simulink model "FaultModel"  (R2020b)
settings: Solver=ode4  StartTime=0.0  StopTime=inf  FixedStep=0.001  RelTol=1e-3
PreLoadFcn:
  | filepath  = fileparts(get_param(bdroot, 'FileName'));
  | cd(filepath);
InitFcn:
  | Init
undefined symbols (not defined in the file): d_i, Earth, F, h_i, Light, MIL, ModelFailEnable, ModelInit_RPM, ModelParam_BattHoverMinutes, ModelParam_BattHoverThr, ModelParam_envAltitude, ModelParam_GPSEphFinal, ModelParam_GPSEpvFinal, ModelParam_GPSEpvInitial, ModelParam_GPSEpvTimeConstant, ModelParam_GPSFix3DFix, ModelParam_GPSSatsVisible, ModelParam_motorCr, ModelParam_motorJm, ModelParam_motorMinThr, ModelParam_motorT, ModelParam_motorWb, ModelParam_noiseGPSSampTime, ModelParam_noiseLowPassFilterCoeAccel, ModelParam_noiseLowPassFilterCoeGyro, ModelParam_noisePowerIMU, ModelParam_noisePowerOffGainAccel, ModelParam_noisePowerOffGainAccelZ, ModelParam_noisePowerOffGainGyro, ModelParam_noisePowerOffGainGyroZ, ModelParam_noisePowerOffGainMag, ModelParam_noisePowerOffGainMagZ, ModelParam_noisePowerOnGainAccel, ModelParam_noisePowerOnGainAccelZ, ModelParam_noisePowerOnGainGyro, ModelParam_noisePowerOnGainGyroZ, ModelParam_noisePowerOnGainMag, ModelParam_noisePowerOnGainMagZ, ModelParam_noiseSampleTimeAccel, ModelParam_noiseSampleTimeGyro, ModelParam_noiseSampleTimeMag, ModelParam_rotorCm, ModelParam_rotorCt, ModelParam_timeSampBaro, ModelParam_uavCCm, ModelParam_uavCd, ModelParam_uavDearo, ModelParam_uavJ, ModelParam_uavMass, ModelParam_uavMotNumbs, ModelParam_uavR, ModelParam_uavType, Moderate, Newton, Raphson, WGS84
libraries: simulink x12, aerolibwind2 x3, aerolibtransform2 x3, sharedtransform x3, aerolibasang x3, aerolibatmos2 x2, aerolibutil x2, shared6dof x1, aerolibconvert2 x1, aerolibobsolete x1, aerolibnav x1, aerolibgravity2 x1
(part 1 of 4)
settings Model: Creator=Jinrui  LastModifiedBy=DELL
settings DataIOCC: ReturnWorkspaceOutputs=off
settings OptimizationCC: ZeroExternalMemoryAtStartup=off  ZeroInternalMemoryAtStartup=off  EfficientTunableParamExpr=on
settings DebuggingCC: ParameterTunabilityLossMsg=error  ArithmeticOperatorsInVariantConditions=warning
settings SFSimCC: SimUseLocalCustomCode=off  MATLABDynamicMemAlloc=off  CustomCodeUndefinedFunction=UseInterfaceOnly  SimTargetLang=C++
settings RTWCC: Description=Embedded Coder  SystemTargetFile=ert.tlc  GenerateMakefile=off  PackageGeneratedCodeAndArtifacts=on  PackageName=MulticopterModel  TemplateMakefile=ert_default_tmf  RTWUseLocalCustomCode=off  TargetLang=C++  RTWCompilerOptimization=on
settings CodeAppCC: ForceParamTrailComments=on  OperatorAnnotations=on  SimulinkDataObjDesc=on  SFDataObjDesc=on  MATLABFcnDesc=on  InsertBlockDesc=on  StateflowObjectComments=on  MATLABSourceComments=on
settings ERTTargetCC: TargetLangStandard=C++03 (ISO)  MultiwordLength=2048  GenerateSampleERTMain=on  CodeInterfacePackaging=C++ class  SupportContinuousTime=on  MultiInstanceErrorCode=None  RootIOFormat=Structure reference  ERTCustomFileTemplate=example_file_process.tlc  ERTFilePackagingFormat=Compact
settings SimscapeCC: SimscapeNormalizeSystem=off

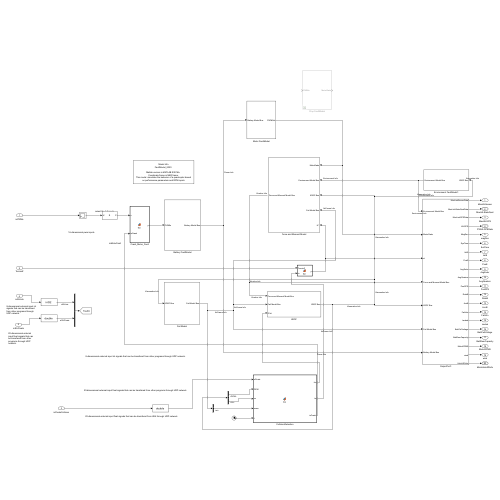
[thumbnail: Simulink's stored preview of the top-level diagram]
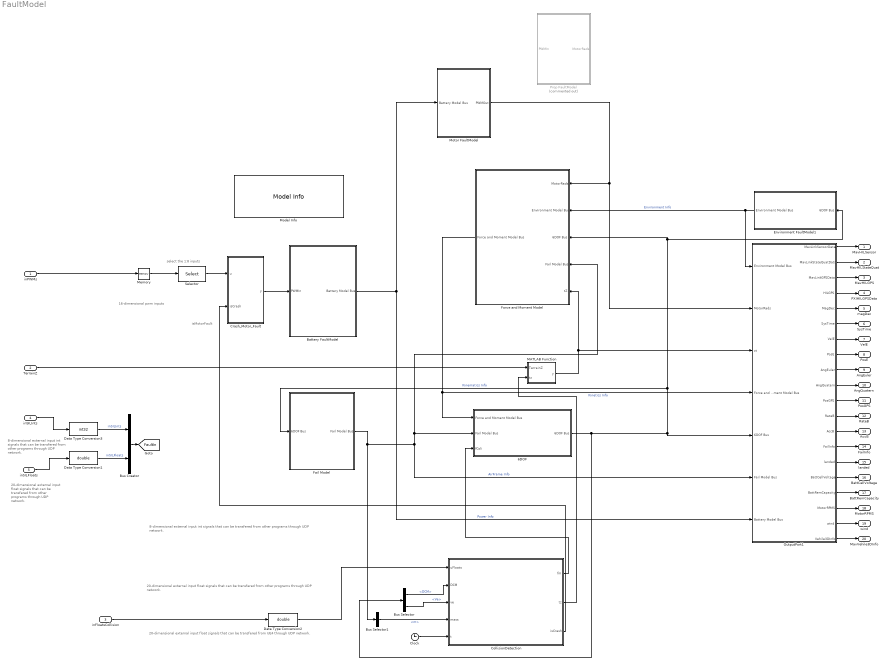
== system FaultModel ==
  note: 16-dimensional pwm inputs
  note: 20-dimensional external input float signals that can be transfered from UE4 through UDP network.
  note: select the 1:8 inputs
  note: 8-dimensional external input int signals that can be transfered from other programs through UDP network.
  note: 20-dimensional external input float signals that can be transfered from other programs through UDP network.
  note: isMotorFault
  note: 20-dimensional external input float signals that can be transfered from other programs through UDP network.
  note: 8-dimensional external input int signals that can be transfered from other programs through UDP network.
  inPWMs : Inport  PortDimensions=8
  TerrainZ : Inport  Port=2  PortDimensions=1
  inFloatsCollision : Inport  Port=3  OutDataTypeStr=single  PortDimensions=20
  inSILInts : Inport  Port=4  OutDataTypeStr=int32  PortDimensions=8
  inSILFloats : Inport  Port=5  OutDataTypeStr=single  PortDimensions=20
  6DOF : Subsystem
  Battery FaultModel : Subsystem
  Bus Creator : BusCreator  Inputs=2
  Bus Selector : BusSelector  OutputSignals=DCM,Ve
  Bus Selector1 : BusSelector  OutputSignals=m
  Clock : Clock
  CollisionDetection : MATLAB Function  TreatAsAtomicUnit=on
  Crash_Motor_Fault : MATLAB Function  TreatAsAtomicUnit=on
  Data Type Conversion1 : DataTypeConversion  OutDataTypeStr=double
  Data Type Conversion2 : DataTypeConversion  OutDataTypeStr=double
  Data Type Conversion3 : DataTypeConversion  OutDataTypeStr=int32
  Environment FaultModel1 : Subsystem
  Fail Model : Subsystem
  Force and Moment Model : Subsystem
  MATLAB Function : MATLAB Function  TreatAsAtomicUnit=on
  Memory : Memory
  Model Info : simulink/Model-Wide Utilities/Model Info  Frame=on  DisplayStringWithTags=|  HorizontalTextAlignment=Center  LeftAlignmentValue=0.5
      | Model Info
      | %<ModelName> 
      | %<Description>   
      | Matlab version is MATLAB R2016b. 
      | Coordinate frame is NED frame.
      |  This model  simulates the behavior of a quadcopter based 
      | on performance parameters and RPM inputs
  Motor FaultModel : Subsystem
  OutputPort1 : Subsystem
  Prop FaultModel : Subsystem  Commented=on
  Selector : Selector  InputPortWidth=8  IndexOptions=Index vector (dialog)  Indices=[1:8]  OutputSizes=1
  MavHILSensor : Outport
  MavHILStateQuat : Outport  Port=2  OutDataTypeStr=Bus: MavLinkStateQuat  VectorParamsAs1DForOutWhenUnconnected=off
  MavHILGPS : Outport  Port=3
  PXIHILGPSData : Outport  Port=4  OutDataTypeStr=Bus: HILGPS  VectorParamsAs1DForOutWhenUnconnected=off
  magDec : Outport  Port=5  VectorParamsAs1DForOutWhenUnconnected=off
  SysTime : Outport  Port=6  VectorParamsAs1DForOutWhenUnconnected=off
  VelE : Outport  Port=7  VectorParamsAs1DForOutWhenUnconnected=off
  PosE : Outport  Port=8  VectorParamsAs1DForOutWhenUnconnected=off
  AngEuler : Outport  Port=9  VectorParamsAs1DForOutWhenUnconnected=off
  AngQuatern : Outport  Port=10  VectorParamsAs1DForOutWhenUnconnected=off
  PosGPS : Outport  Port=11  VectorParamsAs1DForOutWhenUnconnected=off
  RateB : Outport  Port=12  VectorParamsAs1DForOutWhenUnconnected=off
  AccB : Outport  Port=13  VectorParamsAs1DForOutWhenUnconnected=off
  FailInfo : Outport  Port=14  VectorParamsAs1DForOutWhenUnconnected=off
  landed : Outport  Port=15  VectorParamsAs1DForOutWhenUnconnected=off
  BattCellVoltage : Outport  Port=16  VectorParamsAs1DForOutWhenUnconnected=off
  BattRemCapacity : Outport  Port=17  VectorParamsAs1DForOutWhenUnconnected=off
  MotorRPMS : Outport  Port=18  VectorParamsAs1DForOutWhenUnconnected=off
  wind : Outport  Port=19  VectorParamsAs1DForOutWhenUnconnected=off
  MavVehile3DInfo : Outport  Port=20  OutDataTypeStr=Bus: MavVehileInfo  VectorParamsAs1DForOutWhenUnconnected=off
  tag scope: FaultIn=global
  wires:
  OutputPort1/14(FailInfo) -> FailInfo/1
  OutputPort1/9(AngEuler) -> AngEuler/1
  OutputPort1/17(BattRemCapacity) -> BattRemCapacity/1
  Memory/1 -> Selector/1
  OutputPort1/1(MavLinkSensorData) -> MavHILSensor/1
  Force and Moment Model/1(Force and Moment Model Bus) -> 6DOF/1(Force and Moment Model Bus), OutputPort1/4(Force and Moment Model Bus)  "Kinetics Info"
  Battery FaultModel/1(Battery Model Bus) -> Motor FaultModel/1(Battery Model Bus), OutputPort1/7(Battery Model Bus)  "Power Info"
  Fail Model/1(Fail Model Bus) -> Bus Selector1/1, Force and Moment Model/4(Fail Model Bus), 6DOF/2(Fail Model Bus), OutputPort1/6(Fail Model Bus)  "AirFrame Info"
  Bus Selector1/1 -> CollisionDetection/4(mass)  "<m>"
  OutputPort1/15(landed) -> landed/1
  TerrainZ/1 -> MATLAB Function/1(TerrainZ)
  OutputPort1/8(PosE) -> PosE/1
  OutputPort1/19(wind) -> wind/1
  Environment FaultModel1/1(Environment Model Bus) -> OutputPort1/1(Environment Model Bus), Force and Moment Model/2(Environment Model Bus)  "Environment Info"
  inFloatsCollision/1 -> Data Type Conversion2/1
  Bus Selector/1 -> CollisionDetection/2(DCM)  "<DCM>"
  inPWMs/1 -> Memory/1
  MATLAB Function/1(y) -> Force and Moment Model/5("tZ "), OutputPort1/3(zt)
  CollisionDetection/2(tz) -> MATLAB Function/2(tz)
  OutputPort1/10(AngQuatern) -> AngQuatern/1
  OutputPort1/7(VelE) -> VelE/1
  OutputPort1/13(AccB) -> AccB/1
  6DOF/1(6DOF Bus) -> Bus Selector/1, Force and Moment Model/3(6DOF Bus), Environment FaultModel1/1(6DOF Bus), Fail Model/1(6DOF Bus), OutputPort1/5(6DOF Bus)  "Kinematics Info"
  OutputPort1/12(RateB) -> RateB/1
  OutputPort1/5(MagDec) -> magDec/1
  CollisionDetection/1(fm) -> 6DOF/3(fColi)
  OutputPort1/18(MotorRPMS) -> MotorRPMS/1
  OutputPort1/16(BattCellVoltage) -> BattCellVoltage/1
  OutputPort1/20(Vehile3DInfo) -> MavVehile3DInfo/1
  CollisionDetection/3(isCrash) -> Crash_Motor_Fault/2(isCrash)
  Bus Selector/2 -> CollisionDetection/3(ve)  "<Ve>"
  OutputPort1/2(MavLinkStateQuatData) -> MavHILStateQuat/1
  OutputPort1/3(MavLinkGPSData) -> MavHILGPS/1
  Data Type Conversion2/1 -> CollisionDetection/1(uFloats)
  OutputPort1/6(SysTime) -> SysTime/1
  OutputPort1/4(HILGPS) -> PXIHILGPSData/1
  OutputPort1/11(PosGPS) -> PosGPS/1
  Clock/1 -> CollisionDetection/5(t)
  Selector/1 -> Crash_Motor_Fault/1(u)
  Data Type Conversion3/1 -> Bus Creator/1  "inSILInts"
  inSILFloats/1 -> Data Type Conversion1/1
  inSILInts/1 -> Data Type Conversion3/1
  Data Type Conversion1/1 -> Bus Creator/2  "inSILFloats"
  Bus Creator/1 -> [FaultIn]
  Crash_Motor_Fault/1(y) -> Battery FaultModel/1(PWMIn)
  Motor FaultModel/1(PWMOut) -> OutputPort1/2(MotorRads), Force and Moment Model/1(MotorRads)

== system FaultModel/6DOF ==
  Force and Moment Model Bus : Inport
  Fail Model Bus : Inport  Port=2
  fColi : Inport  Port=3
  Bus Creator : BusCreator  Inputs=8
  Bus Selector : BusSelector  OutputSignals=dM,m,J
  Bus Selector1 : BusSelector  OutputSignals=Fb,Mb
  Constant_dI/dt : Constant  Value=zeros(3,3)
  Custom Variable Mass 6DOF (Quaternion) : shared6dof/6DOF (Euler Angles)  units=Metric (MKS)  mtype=Custom Variable  rep=Quaternion  xme_0=ModelInit_PosE  Vm_0=ModelInit_VelB  eul_0=ModelInit_AngEuler  pm_0=ModelInit_RateB  mass_0=1.0  mass_e=0.5  mass_f=2.0  inertia=eye(3)  inertia_e=eye(3)  inertia_f=2*eye(3)  k_quat=1.0  vre_flag=off  abi_flag=off  aMode=aMode  xme_statename=''  Vm_statename=''  eul_statename=''  quat_statename=''  pm_statename=''  mass_statename=''
      settings: SourceProductBaseCode=AE,PW,MT,UV,VE,VP
  Demux : Demux  Outputs=2
  Sum : Sum  Inputs=+++
  Sum1 : Sum  Inputs=++|
  6DOF Bus : Outport  VectorParamsAs1DForOutWhenUnconnected=off
  wires:
  Bus Selector1/1 -> Sum1/2  "<Fb>"
  Bus Selector/2 -> Custom Variable Mass 6DOF (Quaternion)/3  "<m>"
  Custom Variable Mass 6DOF (Quaternion)/8 -> Bus Creator/8  "AccB"
  Sum/1 -> Custom Variable Mass 6DOF (Quaternion)/2
  Constant_dI/dt/1 -> Custom Variable Mass 6DOF (Quaternion)/4
  Custom Variable Mass 6DOF (Quaternion)/5 -> Bus Creator/5  "Vb"
  Custom Variable Mass 6DOF (Quaternion)/6 -> Bus Creator/6  "wb"
  Custom Variable Mass 6DOF (Quaternion)/1 -> Bus Creator/1  "Ve"
  Custom Variable Mass 6DOF (Quaternion)/4 -> Bus Creator/4  "DCM"
  Custom Variable Mass 6DOF (Quaternion)/2 -> Bus Creator/2  "Xe"
  Custom Variable Mass 6DOF (Quaternion)/3 -> Bus Creator/3  "Eular(rad)"
  Custom Variable Mass 6DOF (Quaternion)/7 -> Bus Creator/7  "dwb/dt"
  Bus Selector/3 -> Custom Variable Mass 6DOF (Quaternion)/5  "<J>"
  Bus Selector/1 -> Sum/2  "<dM>"
  Bus Selector1/2 -> Sum/1  "<Mb>"
  Fail Model Bus/1 -> Bus Selector/1
  Force and Moment Model Bus/1 -> Bus Selector1/1
  Bus Creator/1 -> 6DOF Bus/1
  Sum1/1 -> Custom Variable Mass 6DOF (Quaternion)/1
  Demux/1 -> Sum1/1
  fColi/1 -> Demux/1
  Demux/2 -> Sum/3

== system FaultModel/Battery FaultModel ==
  PWMIn : Inport
  FaultModelTmp : Subsystem
  Battery Model Bus : Outport  VectorParamsAs1DForOutWhenUnconnected=off
  wires:
  [FaultIn] -> FaultModelTmp/1(FaultIn)
  PWMIn/1 -> FaultModelTmp/2(PWMIn)
  FaultModelTmp/1(Battery Model Bus) -> Battery Model Bus/1

== system FaultModel/Environment FaultModel1 ==
  6DOF Bus : Inport
  Env FaultWindModel : Subsystem
  Environment Model Bus : Outport  VectorParamsAs1DForOutWhenUnconnected=off
  wires:
  6DOF Bus/1 -> Env FaultWindModel/1(6DOF Bus)
  [FaultIn] -> Env FaultWindModel/2(FaultIn)
  Env FaultWindModel/1(Environment Model Bus) -> Environment Model Bus/1

== system FaultModel/Fail Model ==
  6DOF Bus : Inport
  Prop FaultModel : Subsystem
  Fail Model Bus : Outport  VectorParamsAs1DForOutWhenUnconnected=off
  wires:
  [FaultIn] -> Prop FaultModel/1(FaultIn)
  Prop FaultModel/1(Fail Model Bus) -> Fail Model Bus/1
  6DOF Bus/1 -> Prop FaultModel/2(6DOF Bus)

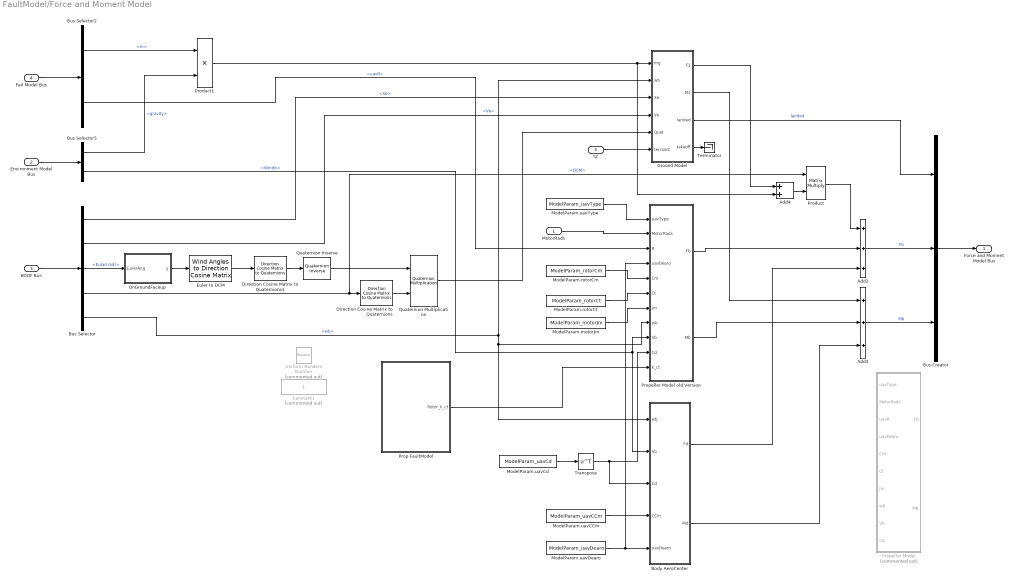
== system FaultModel/Force and Moment Model ==
  MotorRads : Inport
  Environment Model Bus : Inport  Port=2
  6DOF Bus : Inport  Port=3
  Fail Model Bus : Inport  Port=4
  "tZ " : Inport  Port=5
  Add2 : Sum  Inputs=+++
  Add3 : Sum  Inputs=+++
  Add4 : Sum
  Body AeroCenter : MATLAB Function  TreatAsAtomicUnit=on
  Bus Creator : BusCreator  Inputs=3
  Bus Selector : BusSelector  OutputSignals=Xe,Ve,Eular(rad),DCM,wb
  Bus Selector2 : BusSelector  OutputSignals=m,uavR
  Bus Selector5 : BusSelector  OutputSignals=gravity,Windb
  Constant1 : Constant  Commented=on
  Direction Cosine Matrix to Quaternions : sharedtransform/Direction Cosine Matrix  to Quaternions  aMode=aMode  action=None  tolerance=eps(2)
      settings: SourceProductBaseCode=AE,PW,MT,UV,VE,VP
  Direction Cosine Matrix to Quaternions1 : sharedtransform/Direction Cosine Matrix  to Quaternions  aMode=aMode  action=None  tolerance=eps(2)
      settings: SourceProductBaseCode=AE,PW,MT,UV,VE,VP
  Euler to DCM : aerolibtransform2/Wind Angles to  Direction Cosine Matrix
      settings: SourceProductBaseCode=AE
  Ground Model : MATLAB Function  TreatAsAtomicUnit=on
  ModelParam.motorJm : Constant  Value=ModelParam_motorJm
  ModelParam.rotorCm : Constant  Value=ModelParam_rotorCm
  ModelParam.rotorCt : Constant  Value=ModelParam_rotorCt
  ModelParam.uavCCm : Constant  Value=ModelParam_uavCCm
  ModelParam.uavCd : Constant  Value=ModelParam_uavCd
  ModelParam.uavDearo : Constant  Value=ModelParam_uavDearo
  ModelParam.uavType : Constant  Value=ModelParam_uavType
  OnGroundFaceup : MATLAB Function  TreatAsAtomicUnit=on
  Product : Product  Multiplication=Matrix(*)
  Product1 : Product
  Prop FaultModel : Subsystem
  Propeller Model : Subsystem  Commented=on  TreatAsAtomicUnit=on
  Propeller Model old Version : MATLAB Function  TreatAsAtomicUnit=on
  Quaternion Inverse : aerolibutil/Quaternion Inverse
  Quaternion Multiplication : aerolibutil/Quaternion Multiplication
  Terminator : Terminator
  Transpose : Math  Operator=transpose  SignedPower=on  SaturateOnIntegerOverflow=on
  Uniform Random Number : UniformRandomNumber  Commented=on  Minimum=[-1,-1,-1]  Maximum=[1,1,1]  Seed=[145787,351545,2864]  SampleTime=0.05
  Force and Moment Model Bus : Outport  VectorParamsAs1DForOutWhenUnconnected=off
  wires:
  Body AeroCenter/2(Md) -> Add3/3
  Body AeroCenter/1(Fd) -> Add2/3
  Propeller Model old Version/2(Mb) -> Add3/2
  Propeller Model old Version/1(Fb) -> Add2/2
  Ground Model/4(takeoff) -> Terminator/1
  Ground Model/3(landed) -> Bus Creator/1  "landed"
  "tZ "/1 -> Ground Model/6(terrainZ)
  Add3/1 -> Bus Creator/3  "Mb"
  Add2/1 -> Bus Creator/2  "Fb"
  ModelParam.uavType/1 -> Propeller Model old Version/1(uavType)
  Quaternion Multiplication/1 -> Ground Model/5(Quet)
  Quaternion Inverse/1 -> Quaternion Multiplication/1
  Direction Cosine Matrix to Quaternions1/1 -> Quaternion Inverse/1
  Euler to DCM/1 -> Direction Cosine Matrix to Quaternions1/1
  OnGroundFaceup/1(y) -> Euler to DCM/1
  Direction Cosine Matrix to Quaternions/1 -> Quaternion Multiplication/2
  ModelParam.rotorCt/1 -> Propeller Model old Version/6(Ct)
  Product/1 -> Add2/1
  Ground Model/1(F1) -> Add4/1
  Add4/1 -> Product/2
  Product1/1 -> Ground Model/1(mg), Add4/2
  Ground Model/2(M1) -> Add3/1
  Bus Selector/4 -> Direction Cosine Matrix to Quaternions/1, Product/1  "<DCM>"
  ModelParam.motorJm/1 -> Propeller Model old Version/7(Jm)
  ModelParam.rotorCm/1 -> Propeller Model old Version/5(Cm)
  MotorRads/1 -> Propeller Model old Version/2(MotorRads)
  Bus Selector/5 -> Propeller Model old Version/8(wb), Body AeroCenter/1(wb), Ground Model/2(wb)  "<wb>"
  ModelParam.uavCCm/1 -> Body AeroCenter/4(CCm)
  Bus Creator/1 -> Force and Moment Model Bus/1
  6DOF Bus/1 -> Bus Selector/1
  Bus Selector/2 -> Ground Model/4(Ve)  "<Ve>"
  Bus Selector/1 -> Ground Model/3(Xe)  "<Xe>"
  Bus Selector/3 -> OnGroundFaceup/1(EulerAng)  "<Eular(rad)>"
  Bus Selector2/1 -> Product1/1  "<m>"
  Bus Selector5/1 -> Product1/2  "<gravity>"
  Fail Model Bus/1 -> Bus Selector2/1
  Environment Model Bus/1 -> Bus Selector5/1
  Bus Selector2/2 -> Propeller Model old Version/3(R)  "<uavR>"
  Bus Selector5/2 -> Body AeroCenter/2(Vb), Propeller Model old Version/9(Vb)  "<Windb>"
  ModelParam.uavDearo/1 -> Propeller Model old Version/4(uavDearo), Body AeroCenter/5(uavDearo)
  ModelParam.uavCd/1 -> Transpose/1
  Transpose/1 -> Body AeroCenter/3(Cd), Propeller Model old Version/10(Cd)
  Prop FaultModel/1(Rotor_k_ct) -> Propeller Model old Version/11(k_ct)

== system FaultModel/Motor FaultModel ==
  Battery Model Bus : Inport
  Bus Selector : BusSelector  OutputSignals=PWMOut
  FaultModelTmp : Subsystem
  PWMOut : Outport
  wires:
  Battery Model Bus/1 -> Bus Selector/1
  [FaultIn] -> FaultModelTmp/1(FaultIn)
  FaultModelTmp/1(PWMOut) -> PWMOut/1
  Bus Selector/1 -> FaultModelTmp/2(PWMIn)  "<PWMOut>"

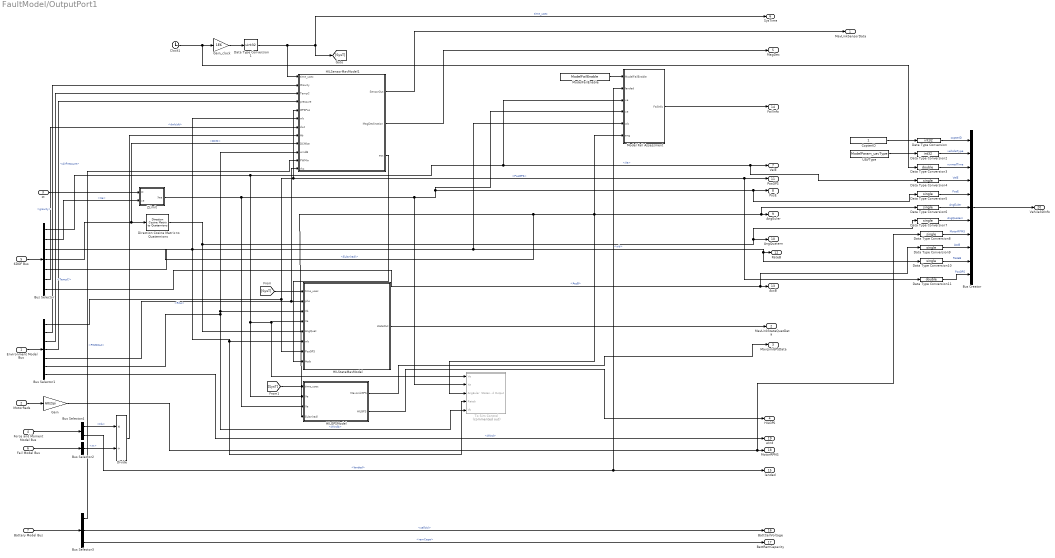
== system FaultModel/OutputPort1 ==
  Environment Model Bus : Inport
  MotorRads : Inport  Port=2
  zt : Inport  Port=3
  Force and Moment Model Bus : Inport  Port=4
  6DOF Bus : Inport  Port=5
  Fail Model Bus : Inport  Port=6
  Battery Model Bus : Inport  Port=7
  Bus Creator : BusCreator  Inputs=11  OutDataTypeStr=Bus: MavVehileInfo
  Bus Selector : BusSelector  OutputSignals=Ve,Xe,Eular(rad),DCM,wb,dwb/dt,AccB
  Bus Selector1 : BusSelector  OutputSignals=PosGPS,gravity,TempC,AirPressure,Rho,Windb,Wind
  Bus Selector2 : BusSelector  OutputSignals=m
  Bus Selector3 : BusSelector  OutputSignals=PWMOut,cellVol,remCapa
  Bus Selector4 : BusSelector  OutputSignals=Fb,landed
  Clock1 : Clock
  CopterID : Constant
  Data Type Conversion : DataTypeConversion  OutDataTypeStr=int32
  Data Type Conversion1 : DataTypeConversion  OutDataTypeStr=uint32
  Data Type Conversion{4..10} (7 alike) : DataTypeConversion  OutDataTypeStr=single
  Data Type Conversion11 : DataTypeConversion  OutDataTypeStr=double
  Data Type Conversion2 : DataTypeConversion  OutDataTypeStr=int32
  Data Type Conversion3 : DataTypeConversion  OutDataTypeStr=double
  Direction Cosine Matrix to Quaternions : sharedtransform/Direction Cosine Matrix  to Quaternions  aMode=aMode  action=None  tolerance=eps(2)
      settings: SourceProductBaseCode=AE,PW,MT,UV,VE,VP
  Divide : Product  Inputs=*/
  Gain : Gain  Gain=60/2/pi
  Gain_clock : Gain  Gain=1E6
  HILGPSModel : Subsystem
  HILSensorMavModel1 : Subsystem
  HILStateMavModel : Subsystem
  Model Fail Assessment : MATLAB Function  TreatAsAtomicUnit=on
  ModelFailEnable : Constant  Value=ModelFailEnable
  To Sim Control : Subsystem  Commented=on
  UAVType : Constant  Value=ModelParam_uavType
  ZLimit : MATLAB Function  TreatAsAtomicUnit=on
  MavLinkSensorData : Outport  VectorParamsAs1DForOutWhenUnconnected=off
  MavLinkStateQuatData : Outport  Port=2  VectorParamsAs1DForOutWhenUnconnected=off
  MavLinkGPSData : Outport  Port=3  VectorParamsAs1DForOutWhenUnconnected=off
  HILGPS : Outport  Port=4  VectorParamsAs1DForOutWhenUnconnected=off
  MagDec : Outport  Port=5  VectorParamsAs1DForOutWhenUnconnected=off
  SysTime : Outport  Port=6  VectorParamsAs1DForOutWhenUnconnected=off
  VelE : Outport  Port=7  VectorParamsAs1DForOutWhenUnconnected=off
  PosE : Outport  Port=8  VectorParamsAs1DForOutWhenUnconnected=off
  AngEuler : Outport  Port=9  VectorParamsAs1DForOutWhenUnconnected=off
  AngQuatern : Outport  Port=10  VectorParamsAs1DForOutWhenUnconnected=off
  PosGPS : Outport  Port=11  VectorParamsAs1DForOutWhenUnconnected=off
  RateB : Outport  Port=12  VectorParamsAs1DForOutWhenUnconnected=off
  AccB : Outport  Port=13  VectorParamsAs1DForOutWhenUnconnected=off
  FailInfo : Outport  Port=14  VectorParamsAs1DForOutWhenUnconnected=off
  landed : Outport  Port=15  VectorParamsAs1DForOutWhenUnconnected=off
  BattCellVoltage : Outport  Port=16  VectorParamsAs1DForOutWhenUnconnected=off
  BattRemCapacity : Outport  Port=17  VectorParamsAs1DForOutWhenUnconnected=off
  MotorRPMS : Outport  Port=18  VectorParamsAs1DForOutWhenUnconnected=off
  wind : Outport  Port=19  VectorParamsAs1DForOutWhenUnconnected=off
  Vehile3DInfo : Outport  Port=20  VectorParamsAs1DForOutWhenUnconnected=off
  wires:
  [SysT] -> HILGPSModel/1(time_usec)
  [SysT] -> HILStateMavModel/1(time_usec)
  Bus Selector/5 -> HILSensorMavModel1/6(wb), Data Type Conversion10/1, RateB/1, Model Fail Assessment/5(wb), To Sim Control/4(Rateb), HILStateMavModel/6(wb)  "<wb>"
  Bus Selector/4 -> HILSensorMavModel1/9(DCMbe), Direction Cosine Matrix to Quaternions/1  "<DCM>"
  Bus Selector/1 -> HILGPSModel/2(Ve), To Sim Control/1(Ve), HILStateMavModel/4(Ve), Model Fail Assessment/3(ve), Data Type Conversion4/1, VelE/1  "<Ve>"
  Bus Selector/6 -> HILSensorMavModel1/7(dwt)  "<dwb/dt>"
  Bus Selector/3 -> Data Type Conversion6/1, AngEuler/1, Model Fail Assessment/6(ang), To Sim Control/3(AngEuler), HILGPSModel/4(Eular(rad))  "<Eular(rad)>"
  Clock1/1 -> Data Type Conversion3/1, Gain_clock/1
  Data Type Conversion1/1 -> HILSensorMavModel1/1(time_usec), SysTime/1, [SysT]  "time_usec"
  Gain_clock/1 -> Data Type Conversion1/1
  6DOF Bus/1 -> Bus Selector/1
  zt/1 -> ZLimit/1(zt)
  Bus Selector/2 -> ZLimit/2(xe)  "<Xe>"
  Environment Model Bus/1 -> Bus Selector1/1
  Bus Selector1/1 -> HILStateMavModel/7(PosGPS), HILSensorMavModel1/5(GPSPos), Data Type Conversion11/1, PosGPS/1  "<PosGPS>"
  Bus Selector1/2 -> HILSensorMavModel1/2(Gravity)  "<gravity>"
  Bus Selector1/3 -> HILSensorMavModel1/3(TempC)  "<TempC>"
  Bus Selector1/4 -> HILSensorMavModel1/4(pressure)  "<AirPressure>"
  Bus Selector1/5 -> HILSensorMavModel1/12(rho), HILStateMavModel/2(pho)  "<Rho>"
  Bus Selector1/6 -> HILSensorMavModel1/10(windB), HILStateMavModel/3(Vb), To Sim Control/5(Vb)  "<Windb>"
  Bus Selector2/1 -> Divide/2  "<m>"
  Bus Selector4/1 -> Divide/1  "<Fb>"
  Force and Moment Model Bus/1 -> Bus Selector4/1
  Fail Model Bus/1 -> Bus Selector2/1
  Bus Selector4/2 -> landed/1, Model Fail Assessment/2(landed)  "<landed>"
  Battery Model Bus/1 -> Bus Selector3/1
  Bus Selector3/2 -> BattCellVoltage/1  "<cellVol>"
  Bus Selector3/3 -> BattRemCapacity/1  "<remCapa>"
  Bus Selector3/1 -> HILSensorMavModel1/11(PWMin)  "<PWMOut>"
  Bus Selector1/7 -> wind/1  "<Wind>"
  MotorRads/1 -> Gain/1
  HILSensorMavModel1/1(SensorOut) -> MavLinkSensorData/1
  HILSensorMavModel1/2(MagDeclination) -> MagDec/1
  Model Fail Assessment/1(FailInfo) -> FailInfo/1
  ZLimit/1(Xee) -> Data Type Conversion5/1, PosE/1, Model Fail Assessment/4(xe), To Sim Control/2(Xe), HILGPSModel/3(Xe)
  Direction Cosine Matrix to Quaternions/1 -> Data Type Conversion7/1, AngQuatern/1, HILStateMavModel/5(AngQuat)
  Divide/1 -> HILSensorMavModel1/8(Ab)
  HILStateMavModel/1(stateOut) -> MavLinkStateQuatData/1
  HILGPSModel/1(MavLinkGPS) -> MavLinkGPSData/1
  HILGPSModel/2(HILGPS) -> HILGPS/1
  Gain/1 -> Data Type Conversion8/1, MotorRPMS/1
  Bus Selector/7 -> Data Type Conversion9/1, AccB/1  "<AccB>"
  CopterID/1 -> Data Type Conversion/1
  Data Type Conversion/1 -> Bus Creator/1  "copterID"
  Data Type Conversion2/1 -> Bus Creator/2  "vehicleType"
  UAVType/1 -> Data Type Conversion2/1
  Data Type Conversion3/1 -> Bus Creator/3  "runnedTime"
  Data Type Conversion4/1 -> Bus Creator/4  "VelE"
  Data Type Conversion5/1 -> Bus Creator/5  "PosE"
  Data Type Conversion6/1 -> Bus Creator/6  "AngEuler"
  Data Type Conversion7/1 -> Bus Creator/7  "AngQuatern"
  Data Type Conversion8/1 -> Bus Creator/8  "MotorRPMS"
  Data Type Conversion9/1 -> Bus Creator/9  "AccB"
  Data Type Conversion10/1 -> Bus Creator/10  "RateB"
  Data Type Conversion11/1 -> Bus Creator/11  "PosGPS"
  HILSensorMavModel1/3(acc) -> HILStateMavModel/8(Accb)
  ModelFailEnable/1 -> Model Fail Assessment/1(ModelFailEnable)
  Bus Creator/1 -> Vehile3DInfo/1

== system FaultModel/Prop FaultModel ==
  PWMIn : Inport
  Prop FaultModel : Subsystem
  MotorRads : Outport  VectorParamsAs1DForOutWhenUnconnected=off
  wires:
  Prop FaultModel/1(PWMOut) -> MotorRads/1
  [FaultIn] -> Prop FaultModel/1(FaultIn)
  PWMIn/1 -> Prop FaultModel/2(PWMIn)

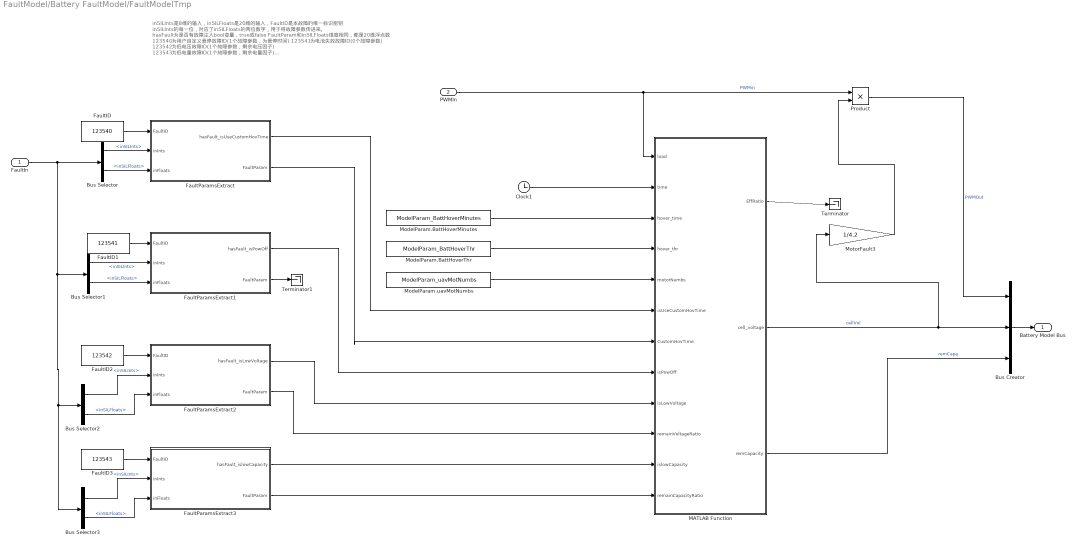
== system FaultModel/Battery FaultModel/FaultModelTmp ==
  note: inSILInts是8维的输入，inSILFloats是20维的输入，FaultID是本故障的唯一标识密钥
      | inSILInts的每一位，对应了inSILFloats的两位数字，用于将故障参数传进来。
      |
      | hasFault为是否有故障注入bool变量，true或false
      | FaultParam和inSILFloats维度相同，都是20维浮点数
      |
      | 123540为用户自定义悬停故障ID(1个故障参数，为悬停时间)
      | 123541为电池失效故障ID(0个故障参数)
      | 123542为低电压故障ID(1个故障参数，剩余电压因子)
      | 123543为低电量故障ID(1个故障参数，剩余电量因子)
      |
      | 注：如果没有新的故障注入进来，FaultParamsExtract会保持上一时刻的值。
  FaultIn : Inport
  PWMIn : Inport  Port=2
  Bus Creator : BusCreator  Inputs=3
  Bus Selector{,1..3} (4 alike) : BusSelector  OutputSignals=inSILInts,inSILFloats
  Clock1 : Clock
  FaultID : Constant  Value=123540  OutDataTypeStr=int32
  FaultID1 : Constant  Value=123541  OutDataTypeStr=int32
  FaultID2 : Constant  Value=123542  OutDataTypeStr=int32
  FaultID3 : Constant  Value=123543  OutDataTypeStr=int32
  FaultParamsExtract : MATLAB Function  TreatAsAtomicUnit=on
  FaultParamsExtract1 : MATLAB Function  TreatAsAtomicUnit=on
  FaultParamsExtract2 : MATLAB Function  TreatAsAtomicUnit=on
  FaultParamsExtract3 : MATLAB Function  TreatAsAtomicUnit=on
  MATLAB Function : MATLAB Function  TreatAsAtomicUnit=on  SystemSampleTime=0.01
  ModelParam.BattHoverMinutes : Constant  Value=ModelParam_BattHoverMinutes
  ModelParam.BattHoverThr : Constant  Value=ModelParam_BattHoverThr
  ModelParam.uavMotNumbs : Constant  Value=ModelParam_uavMotNumbs
  MotorFault3 : Gain  Gain=1/4.2
  Product : Product
  Terminator : Terminator
  Terminator1 : Terminator
  Battery Model Bus : Outport  VectorParamsAs1DForOutWhenUnconnected=off
  wires:
  FaultID/1 -> FaultParamsExtract/1(FaultID)
  FaultParamsExtract2/2(FaultParam) -> MATLAB Function/10(remainVoltageRatio)
  FaultParamsExtract1/1(hasFault_isPowOff) -> MATLAB Function/8(isPowOff)
  MATLAB Function/1(EffRatio) -> Terminator/1
  FaultParamsExtract2/1(hasFault_isLowVoltage) -> MATLAB Function/9(isLowVoltage)
  MotorFault3/1 -> Product/2
  PWMIn/1 -> MATLAB Function/1(load), Product/1  "PWMin"
  MATLAB Function/3(remCapacity) -> Bus Creator/3  "remCapa"
  Product/1 -> Bus Creator/1  "PWMOut"
  MATLAB Function/2(cell_voltage) -> MotorFault3/1, Bus Creator/2  "cellVol"
  ModelParam.uavMotNumbs/1 -> MATLAB Function/5(motorNumbs)
  Clock1/1 -> MATLAB Function/2(time)
  FaultParamsExtract3/2(FaultParam) -> MATLAB Function/12(remainCapacityRatio)
  FaultParamsExtract/1(hasFault_isUseCustomHovTime) -> MATLAB Function/6(isUseCustomHovTime)
  FaultParamsExtract/2(FaultParam) -> MATLAB Function/7(CustomHovTime)
  ModelParam.BattHoverThr/1 -> MATLAB Function/4(hover_thr)
  ModelParam.BattHoverMinutes/1 -> MATLAB Function/3(hover_time)
  Bus Creator/1 -> Battery Model Bus/1
  FaultParamsExtract3/1(hasFault_islowCapacity) -> MATLAB Function/11(islowCapacity)
  FaultID1/1 -> FaultParamsExtract1/1(FaultID)
  FaultIn/1 -> Bus Selector3/1, Bus Selector2/1, Bus Selector1/1, Bus Selector/1
  FaultID2/1 -> FaultParamsExtract2/1(FaultID)
  FaultID3/1 -> FaultParamsExtract3/1(FaultID)
  FaultParamsExtract1/2(FaultParam) -> Terminator1/1
  Bus Selector1/1 -> FaultParamsExtract1/2(inInts)  "<inSILInts>"
  Bus Selector1/2 -> FaultParamsExtract1/3(inFloats)  "<inSILFloats>"
  Bus Selector/1 -> FaultParamsExtract/2(inInts)  "<inSILInts>"
  Bus Selector/2 -> FaultParamsExtract/3(inFloats)  "<inSILFloats>"
  Bus Selector2/1 -> FaultParamsExtract2/2(inInts)  "<inSILInts>"
  Bus Selector2/2 -> FaultParamsExtract2/3(inFloats)  "<inSILFloats>"
  Bus Selector3/1 -> FaultParamsExtract3/2(inInts)  "<inSILInts>"
  Bus Selector3/2 -> FaultParamsExtract3/3(inFloats)  "<inSILFloats>"

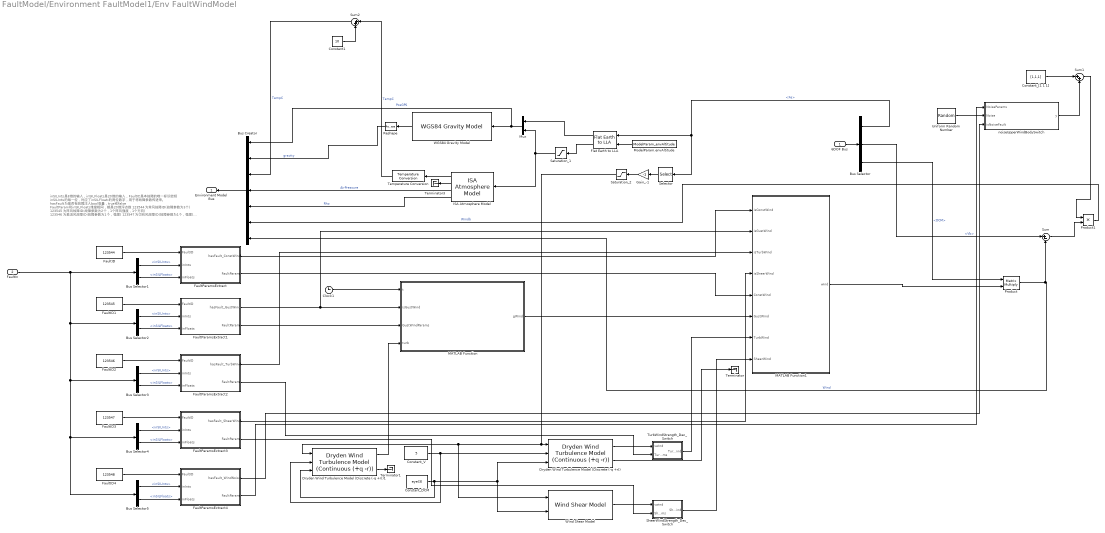
== system FaultModel/Environment FaultModel1/Env FaultWindModel ==
  note: inSILInts是8维的输入，inSILFloats是20维的输入，FaultID是本故障的唯一标识密钥
      | inSILInts的每一位，对应了inSILFloats的两位数字，用于将故障参数传进来。
      |
      | hasFault为是否有故障注入bool变量，true或false
      | FaultParam和inSILFloats维度相同，都是20维浮点数
      |
      | 123544为常风故障ID(故障参数为3个)
      | 123545为阵风故障ID(故障参数为2个，1个阵风强度，1个方向)
      | 123546为紊流风故障ID(故障参数为1个，强度)
      | 123547为切向风故障ID(故障参数为1个，强度)
      | 123548为噪声风故障ID(参数为2个，1格式风振幅扰动因子范围0到1,1个风增益水平）)
      | 注：如果没有新的故障注入进来，FaultParamsExtract会保持上一时刻的值。
  6DOF Bus : Inport
  FaultIn : Inport  Port=2
  Bus Creator : BusCreator  Inputs=7
  Bus Selector : BusSelector  OutputSignals=Xe,Vb,DCM
  Bus Selector{1..5} (5 alike) : BusSelector  OutputSignals=inSILInts,inSILFloats
  Clock1 : Clock
  Constant1 : Constant  Value=10
  Constant_DCM : Constant  Value=eye(3)
  Constant_V : Constant  Value=5
  Constant_[1 1 1] : Constant  Value=[1,1,1]  VectorParams1D=off
  Dryden Wind Turbulence Model (Discrete (-q +r)) : aerolibwind2/Dryden Wind Turbulence Model  (Continuous (+q -r))  units=Metric (MKS)  spec=MIL-F-8785C  model=Discrete Dryden (-q +r)  W20=5  Wdeg=1*1  TurbProb=10^-3 - Moderate  L_high=533.4  Wingspan=1  ts=ModelParam_timeSampTurbWind  Seed=[23341 23342 23343 23344]  T_on=on
  Dryden Wind Turbulence Model (Discrete (-q +r))1 : aerolibwind2/Dryden Wind Turbulence Model  (Continuous (+q -r))  units=Metric (MKS)  spec=MIL-F-8785C  model=Discrete Dryden (-q +r)  W20=2*1  Wdeg=0  TurbProb=10^-2 - Light  L_high=533.4  Wingspan=1  ts=ModelParam_timeSampTurbWind  Seed=[23301 23542 82443 33344]  T_on=on
  FaultID : Constant  Value=123544  OutDataTypeStr=int32
  FaultID1 : Constant  Value=123545  OutDataTypeStr=int32
  FaultID2 : Constant  Value=123546  OutDataTypeStr=int32
  FaultID3 : Constant  Value=123547  OutDataTypeStr=int32
  FaultID4 : Constant  Value=123548  OutDataTypeStr=int32
  FaultParamsExtract : MATLAB Function  TreatAsAtomicUnit=on
  FaultParamsExtract1 : MATLAB Function  TreatAsAtomicUnit=on
  FaultParamsExtract2 : MATLAB Function  TreatAsAtomicUnit=on
  FaultParamsExtract3 : MATLAB Function  TreatAsAtomicUnit=on
  FaultParamsExtract4 : MATLAB Function  TreatAsAtomicUnit=on
  Flat Earth to LLA : aerolibtransform2/Flat Earth to LLA  units=Metric (MKS)  ptype=Earth (WGS84)  F=1/298.257223563  R=6378137  refPosPort=off  LL0=ModelParam_GPSLatLong  psi=0
  Gain_-1 : Gain  Gain=-1
  ISA Atmosphere Model : aerolibatmos2/ISA Atmosphere Model  custom=off  g=9.80665  gamma=1.4  R=287.0531  L=0.0065  h_trop=11000  h_strat=20000  rho0=1.225  P0=101325  T0=288.15  h0=0
  MATLAB Function : MATLAB Function  TreatAsAtomicUnit=on
  MATLAB Function1 : MATLAB Function  TreatAsAtomicUnit=on
  ModelParam.envAltitude : Constant  Value=ModelParam_envAltitude
  Mux : Mux  Inputs=2
  Product : Product  Multiplication=Matrix(*)
  Product1 : Product
  Reshape : Reshape
  Saturation_1 : Saturate  UpperLimit=100000  LowerLimit=0
  Saturation_2 : Saturate  UpperLimit=10000  LowerLimit=0
  Selector : Selector  InputPortWidth=3  IndexOptions=Index vector (dialog)  Indices=[3]  OutputSizes=1
  SheerWindStrength_Dec_Switch : MATLAB Function  TreatAsAtomicUnit=on
  Sum : Sum  Inputs=|+-
  Sum1 : Sum  Inputs=|++
  Sum2 : Sum  Inputs=|++
  Temperature Conversion : aerolibconvert2/Temperature Conversion  IU=K  OU=C
      settings: SourceProductBaseCode=AE
  Terminator : Terminator
  Terminator1 : Terminator
  Terminator3 : Terminator
  TurbWindStrength_Dec_Switch : MATLAB Function  TreatAsAtomicUnit=on
  Uniform Random Number : UniformRandomNumber  Minimum=[-1,-1,-0.5]  Maximum=[1,1,0.5]  Seed=[564565,6846798,46545]  SampleTime=0.003
  "WGS84 Gravity Model " : aerolibobsolete/WGS84 Gravity Model   model=WGS84 Taylor Series  units=Metric (MKS)  no_atmos=on  precessing=on  jd_loc=off  month=October  day=10  year=2004  no_centrifugal=on  action=Warning
      settings: SourceProductBaseCode=AE
  Wind Shear Model : aerolibwind2/Wind Shear Model  units=Metric (MKS)  phase=Category C - Terminal Flight Phase  W_20=2*1  Wdeg=1*1
  noiseUpperWindBodySwitch : MATLAB Function  TreatAsAtomicUnit=on
  Environment Model Bus : Outport  VectorParamsAs1DForOutWhenUnconnected=off
  wires:
  Sum2/1 -> Bus Creator/3  "TempC"
  Bus Selector3/1 -> FaultParamsExtract2/2(inInts)  "<inSILInts>"
  Selector/1 -> Gain_-1/1
  Saturation_2/1 -> Wind Shear Model/1, Dryden Wind Turbulence Model (Discrete (-q +r))1/1, Dryden Wind Turbulence Model (Discrete (-q +r))/1
  noiseUpperWindBodySwitch/1(y) -> Sum1/2
  Constant_DCM/1 -> Dryden Wind Turbulence Model (Discrete (-q +r))/3, Wind Shear Model/2, Dryden Wind Turbulence Model (Discrete (-q +r))1/3
  SheerWindStrength_Dec_Switch/1(SheerWind) -> MATLAB Function1/8(SheerWind)
  FaultParamsExtract1/1(hasFault_GustWind) -> MATLAB Function/2(isGustWind), MATLAB Function1/2(isGustWind)
  Flat Earth to LLA/1 -> Mux/1
  FaultIn/1 -> Bus Selector5/1, Bus Selector4/1, Bus Selector3/1, Bus Selector2/1, Bus Selector1/1
  "WGS84 Gravity Model "/1 -> Reshape/1
  Bus Selector/3 -> Product/1  "<DCM>"
  Bus Selector/1 -> Selector/1, Flat Earth to LLA/1  "<Xe>"
  FaultID2/1 -> FaultParamsExtract2/1(FaultID)
  Bus Selector3/2 -> FaultParamsExtract2/3(inFloats)  "<inSILFloats>"
  FaultParamsExtract3/1(hasFault_SheerWind) -> MATLAB Function1/4(isSheerWind)
  Product1/1 -> Bus Creator/6  "Windb"
  Bus Selector4/1 -> FaultParamsExtract3/2(inInts)  "<inSILInts>"
  ISA Atmosphere Model/4 -> Bus Creator/5  "Rho"
  FaultID1/1 -> FaultParamsExtract1/1(FaultID)
  Mux/1 -> Bus Creator/1, "WGS84 Gravity Model "/1  "PosGPS"
  Constant_V/1 -> Dryden Wind Turbulence Model (Discrete (-q +r))1/2, Dryden Wind Turbulence Model (Discrete (-q +r))/2
  Bus Selector5/2 -> FaultParamsExtract4/3(inFloats)  "<inSILFloats>"
  Bus Selector2/2 -> FaultParamsExtract1/3(inFloats)  "<inSILFloats>"
  FaultID4/1 -> FaultParamsExtract4/1(FaultID)
  Dryden Wind Turbulence Model (Discrete (-q +r))/2 -> Terminator/1
  FaultParamsExtract4/2(FaultParam) -> noiseUpperWindBodySwitch/1(NoiseParams)
  Bus Selector5/1 -> FaultParamsExtract4/2(inInts)  "<inSILInts>"
  FaultParamsExtract4/1(hasFault_WindNoise) -> noiseUpperWindBodySwitch/3(isNoiseFault)
  MATLAB Function1/1(wind) -> Product/2
  ISA Atmosphere Model/2 -> Terminator3/1
  Dryden Wind Turbulence Model (Discrete (-q +r))/1 -> TurbWindStrength_Dec_Switch/1(vwind)
  ISA Atmosphere Model/3 -> Bus Creator/4  "AirPressure"
  ISA Atmosphere Model/1 -> Temperature Conversion/1
  Bus Selector2/1 -> FaultParamsExtract1/2(inInts)  "<inSILInts>"
  Flat Earth to LLA/2 -> Saturation_1/1
  Dryden Wind Turbulence Model (Discrete (-q +r))1/1 -> MATLAB Function/4(turb)
  Dryden Wind Turbulence Model (Discrete (-q +r))1/2 -> Terminator1/1
  Wind Shear Model/1 -> SheerWindStrength_Dec_Switch/1(vwind)
  Clock1/1 -> MATLAB Function/1(t)
  Sum1/1 -> Product1/1
  FaultID/1 -> FaultParamsExtract/1(FaultID)
  6DOF Bus/1 -> Bus Selector/1
  Constant1/1 -> Sum2/2
  Bus Selector/2 -> Sum/1  "<Vb>"
  Temperature Conversion/1 -> Sum2/1  "TempC"
  Bus Creator/1 -> Environment Model Bus/1
  Sum/1 -> Product1/2
  Product/1 -> Bus Creator/7, Sum/2  "Wind"
  Uniform Random Number/1 -> noiseUpperWindBodySwitch/2(Noise)
  Gain_-1/1 -> Saturation_2/1
  Constant_[1 1 1]/1 -> Sum1/1
  Saturation_1/1 -> Mux/2, ISA Atmosphere Model/1
  FaultID3/1 -> FaultParamsExtract3/1(FaultID)
  TurbWindStrength_Dec_Switch/1(TurbWind) -> MATLAB Function1/7(TurbWind)
  Bus Selector4/2 -> FaultParamsExtract3/3(inFloats)  "<inSILFloats>"
  FaultParamsExtract2/1(hasFault_TurbWind) -> MATLAB Function1/3(isTurbWind)
  Reshape/1 -> Bus Creator/2  "gravity"
  Bus Selector1/2 -> FaultParamsExtract/3(inFloats)  "<inSILFloats>"
  ModelParam.envAltitude/1 -> Flat Earth to LLA/2
  FaultParamsExtract1/2(FaultParam) -> MATLAB Function/3(GustWindParams)
  MATLAB Function/1(gWind) -> MATLAB Function1/6(GustWind)
  Bus Selector1/1 -> FaultParamsExtract/2(inInts)  "<inSILInts>"
  FaultParamsExtract2/2(FaultParam) -> TurbWindStrength_Dec_Switch/2(TurbWindParams)
  FaultParamsExtract/1(hasFault_ConstWind) -> MATLAB Function1/1(isConstWind)
  FaultParamsExtract/2(FaultParam) -> MATLAB Function1/5(ConstWind)
  FaultParamsExtract3/2(FaultParam) -> SheerWindStrength_Dec_Switch/2(SheerWindParams)

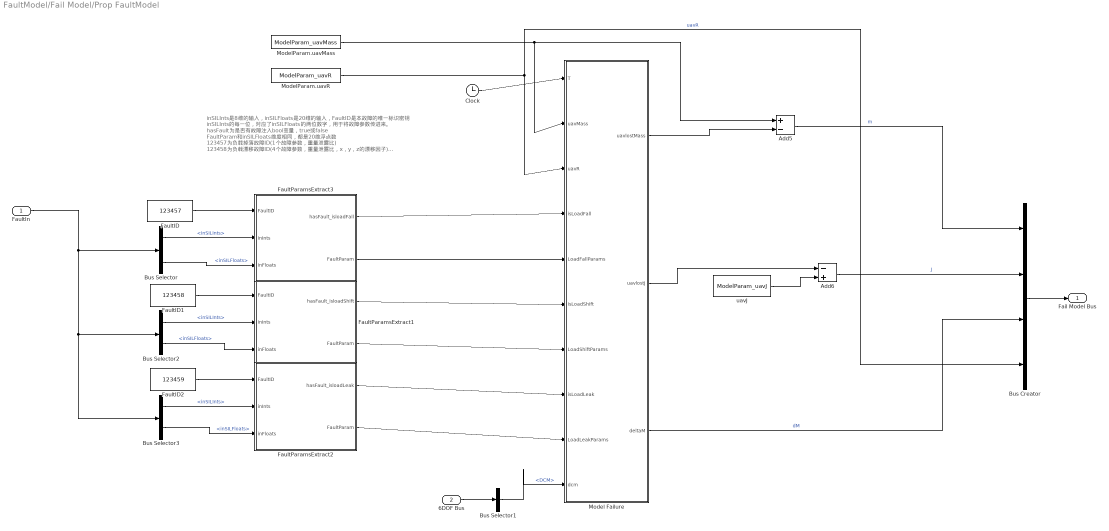
== system FaultModel/Fail Model/Prop FaultModel ==
  note: inSILInts是8维的输入，inSILFloats是20维的输入，FaultID是本故障的唯一标识密钥
      | inSILInts的每一位，对应了inSILFloats的两位数字，用于将故障参数传进来。
      |
      | hasFault为是否有故障注入bool变量，true或false
      | FaultParam和inSILFloats维度相同，都是20维浮点数
      |
      | 123457为负载掉落故障ID(1个故障参数，重量泄露比)
      | 123458为负载漂移故障ID(4个故障参数，重量泄露比，x，y，z的漂移因子)
      | 123459为负载泄露故障ID(2个故障参数，1个重量泄露比，1个泄露因子)
      | 注：如果没有新的故障注入进来，FaultParamsExtract会保持上一时刻的值。
  FaultIn : Inport
  6DOF Bus : Inport  Port=2
  Add5 : Sum  Inputs=+-
  Add6 : Sum  Inputs=-+
  Bus Creator : BusCreator  Inputs=4
  Bus Selector : BusSelector  OutputSignals=inSILInts,inSILFloats
  Bus Selector1 : BusSelector  OutputSignals=DCM
  Bus Selector2 : BusSelector  OutputSignals=inSILInts,inSILFloats
  Bus Selector3 : BusSelector  OutputSignals=inSILInts,inSILFloats
  Clock : Clock
  FaultID : Constant  Value=123457  OutDataTypeStr=int32
  FaultID1 : Constant  Value=123458  OutDataTypeStr=int32
  FaultID2 : Constant  Value=123459  OutDataTypeStr=int32
  FaultParamsExtract1 : MATLAB Function  TreatAsAtomicUnit=on
  FaultParamsExtract2 : MATLAB Function  TreatAsAtomicUnit=on
  FaultParamsExtract3 : MATLAB Function  TreatAsAtomicUnit=on
  Model Failure : MATLAB Function  TreatAsAtomicUnit=on
  ModelParam.uavMass : Constant  Value=ModelParam_uavMass
  ModelParam.uavR : Constant  Value=ModelParam_uavR
  uavJ : Constant  Value=ModelParam_uavJ
  Fail Model Bus : Outport  VectorParamsAs1DForOutWhenUnconnected=off
  wires:
  FaultID/1 -> FaultParamsExtract3/1(FaultID)
  FaultParamsExtract3/1(hasFault_isloadFall) -> Model Failure/4(isLoadFall)
  6DOF Bus/1 -> Bus Selector1/1
  Clock/1 -> Model Failure/1(T)
  Model Failure/2(uavlostJ) -> Add6/1
  Add6/1 -> Bus Creator/2  "J"
  Model Failure/3(deltaM) -> Bus Creator/3  "dM"
  Bus Selector1/1 -> Model Failure/10(dcm)  "<DCM>"
  ModelParam.uavMass/1 -> Model Failure/2(uavMass), Add5/1
  Add5/1 -> Bus Creator/1  "m"
  Model Failure/1(uavlostMass) -> Add5/2
  Bus Creator/1 -> Fail Model Bus/1
  ModelParam.uavR/1 -> Model Failure/3(uavR), Bus Creator/4  "uavR"
  uavJ/1 -> Add6/2
  Bus Selector2/2 -> FaultParamsExtract1/3(inFloats)  "<inSILFloats>"
  Bus Selector2/1 -> FaultParamsExtract1/2(inInts)  "<inSILInts>"
  FaultID1/1 -> FaultParamsExtract1/1(FaultID)
  FaultParamsExtract1/1(hasFault_isloadShift) -> Model Failure/6(isLoadShift)
  FaultParamsExtract1/2(FaultParam) -> Model Failure/7(LoadShiftParams)
  FaultIn/1 -> Bus Selector/1, Bus Selector3/1, Bus Selector2/1
  FaultParamsExtract2/2(FaultParam) -> Model Failure/9(LoadLeakParams)
  FaultParamsExtract3/2(FaultParam) -> Model Failure/5(LoadFallParams)
  FaultID2/1 -> FaultParamsExtract2/1(FaultID)
  FaultParamsExtract2/1(hasFault_isloadLeak) -> Model Failure/8(isLoadLeak)
  Bus Selector3/1 -> FaultParamsExtract2/2(inInts)  "<inSILInts>"
  Bus Selector3/2 -> FaultParamsExtract2/3(inFloats)  "<inSILFloats>"
  Bus Selector/1 -> FaultParamsExtract3/2(inInts)  "<inSILInts>"
  Bus Selector/2 -> FaultParamsExtract3/3(inFloats)  "<inSILFloats>"

== system FaultModel/Force and Moment Model/Prop FaultModel ==
  Prop FaultModel : Subsystem
  Rotor_k_ct : Outport  VectorParamsAs1DForOutWhenUnconnected=off
  wires:
  Prop FaultModel/1(Param_k_ct) -> Rotor_k_ct/1
  [FaultIn] -> Prop FaultModel/1(FaultIn)

== system FaultModel/Force and Moment Model/Propeller Model ==
  uavType : Inport
  MotorRads : Inport  Port=2
  uavR : Inport  Port=3
  uavDearo : Inport  Port=4
  Cm : Inport  Port=5
  Ct : Inport  Port=6
  Jm : Inport  Port=7
  wb : Inport  Port=8
  Vb : Inport  Port=9
  Cd : Inport  Port=10
  Car : Subsystem  TreatAsAtomicUnit=on
  If : If  IfExpression=u1 >= 50
  Multicopter : Subsystem  TreatAsAtomicUnit=on
  Switch : Switch  Threshold=50
  Switch1 : Switch  Threshold=50
  Terminator : Terminator
  Terminator1 : Terminator
  Fb : Outport  VectorParamsAs1DForOutWhenUnconnected=off
  Mb : Outport  Port=2  VectorParamsAs1DForOutWhenUnconnected=off
  wires:
  Vb/1 -> Terminator/1
  Cd/1 -> Terminator1/1
  uavType/1 -> If/1, Switch/2, Switch1/2, Multicopter/1(uavType)
  Switch/1 -> Fb/1
  Switch1/1 -> Mb/1
  If/2 -> Multicopter/Action
  If/1 -> Car/Action
  Car/1(Fb) -> Switch/1
  Multicopter/1(Fb) -> Switch/3
  Car/2(Mb) -> Switch1/1
  Multicopter/2(Mb) -> Switch1/3
  MotorRads/1 -> Car/1(MotorRads), Multicopter/2(MotorRads)
  uavDearo/1 -> Multicopter/4(uavDearo)
  Cm/1 -> Multicopter/5(Cm)
  Ct/1 -> Multicopter/6(Ct)
  Jm/1 -> Multicopter/7(Jm)
  wb/1 -> Multicopter/8(wb)
  uavR/1 -> Multicopter/3(uavR)

== system FaultModel/Motor FaultModel/FaultModelTmp ==
  note: inSILInts是8维的输入，inSILFloats是20维的输入，FaultID是本故障的唯一标识密钥
      | inSILInts的每一位，对应了inSILFloats的两位数字，用于将故障参数传进来。
      |
      | hasFault为是否有故障注入bool变量，true或false
      | FaultParam和inSILFloats维度相同，都是20维浮点数
      |
      | 123450为电机故障ID
      |
      | 注：如果没有新的故障注入进来，FaultParamsExtract会保持上一时刻的值。
  FaultIn : Inport
  PWMIn : Inport  Port=2
  Bus Selector : BusSelector  OutputSignals=inSILInts,inSILFloats
  Bus Selector1 : BusSelector  OutputSignals=inSILInts,inSILFloats
  FaultID : Constant  Value=123450  OutDataTypeStr=int32
  FaultID1 : Constant  Value=123549  OutDataTypeStr=int32
  FaultParamsExtract : MATLAB Function  TreatAsAtomicUnit=on
  FaultParamsExtract1 : MATLAB Function  TreatAsAtomicUnit=on
  MATLAB Function : MATLAB Function  TreatAsAtomicUnit=on
  MotorFaultModel : MATLAB Function  TreatAsAtomicUnit=on
  Motor_Fun : Subsystem
  motor_fauilure_protection : MATLAB Function  TreatAsAtomicUnit=on
  PWMOut : Outport  VectorParamsAs1DForOutWhenUnconnected=off
  wires:
  FaultID/1 -> FaultParamsExtract/1(FaultID)
  FaultParamsExtract/1(hasFault) -> MotorFaultModel/1(hasFault), MATLAB Function/1(isnoMotorProFault)
  FaultParamsExtract/2(FaultParam) -> MotorFaultModel/2(FaultParams)
  Motor_Fun/1(PWMOut) -> PWMOut/1
  FaultID1/1 -> FaultParamsExtract1/1(FaultID)
  FaultParamsExtract1/1(hasFault) -> motor_fauilure_protection/1(hasFault), MATLAB Function/2(isMotorProFault)
  FaultIn/1 -> Bus Selector1/1, Bus Selector/1
  PWMIn/1 -> motor_fauilure_protection/3(inPWMs), MATLAB Function/3(inPWMs), MotorFaultModel/3(inPWMs)
  FaultParamsExtract1/2(FaultParam) -> motor_fauilure_protection/2(FaultParams)
  MATLAB Function/1(y) -> Motor_Fun/1(PWMIn)
  MotorFaultModel/1(y) -> MATLAB Function/4(NoProPWMOut)
  motor_fauilure_protection/1(y) -> MATLAB Function/5(ProPWMOut)
  FaultParamsExtract/3(count) -> MotorFaultModel/4(count)
  FaultParamsExtract1/3(count) -> motor_fauilure_protection/4(count)
  Bus Selector1/1 -> FaultParamsExtract1/2(inInts)  "<inSILInts>"
  Bus Selector1/2 -> FaultParamsExtract1/3(inFloats)  "<inSILFloats>"
  Bus Selector/1 -> FaultParamsExtract/2(inInts)  "<inSILInts>"
  Bus Selector/2 -> FaultParamsExtract/3(inFloats)  "<inSILFloats>"
